simulink model "Modell_PADDELEC_RB_V4"  (R2020a)
settings: Solver=VariableStepAuto  StartTime=0.0  StopTime=250  RelTol=1e-3
values from neighbouring files (symbols this model uses):
  A_s = 3.5    [start.m]
  BAT = clsBattery    [start.m]
  BLDC = clsBLDC    [start.m]
  BoatHull = clsBoatHull    [start.m]
  c_r = 0.003    [start.m]
  MotorECU = clsMotorECU    [start.m]
libraries: fl_lib x54, nesl_utility x28, ee_lib x4, simulink x2, eeGeneralControl x1
settings Model: Creator=Rene Budich  LastModifiedBy=Rene Budich

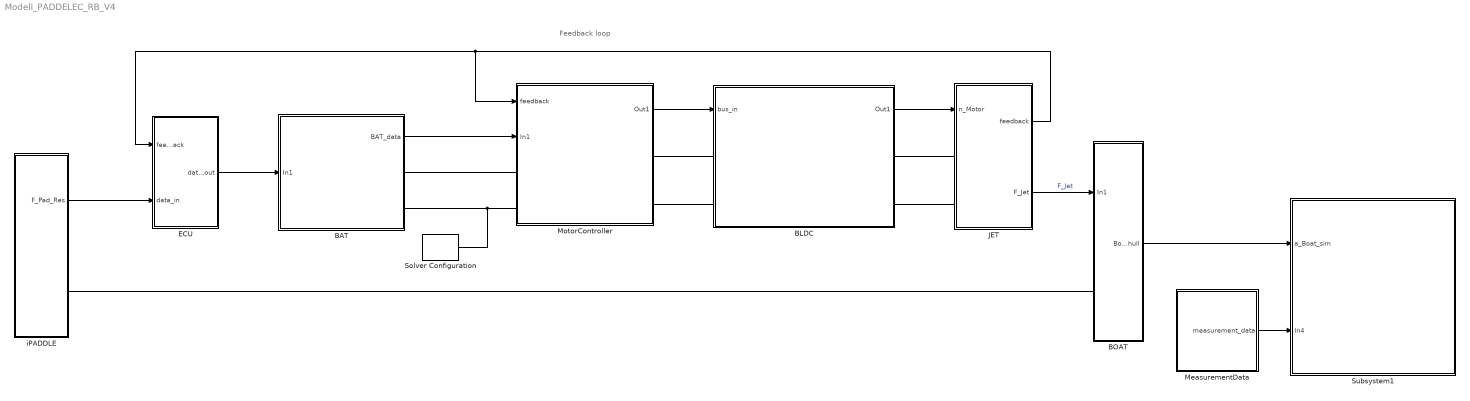
== system Modell_PADDELEC_RB_V4 ==
  note: Feedback loop
  BAT : Subsystem
      mask Display: image('Battery.jpg'); % Use "Edit Image" on toolstrip to change.
  BLDC : Subsystem
      mask Display: image('Motor.png'); % Use "Edit Image" on toolstrip to change.
  BOAT : Subsystem
  ECU : Subsystem
  "JET " : Subsystem
  MeasurementData : Subsystem
  MotorController : Subsystem
      mask Display: image('MotorECU.jpg'); % Use "Edit Image" on toolstrip to change.
  Solver Configuration : nesl_utility/Solver Configuration  PhysicalDomain=network_engine_domain  SubClassName=solver  LeftPortType=input  RightPortType=generic  Tones=[]  Harmonics=[]  SimulateNoise=off  Profile=off  UseLocalSampling=off  EnableSwitchedLinearOptims=on  FrequencyDomain=off  UseCCode=off  RelTol=0.001  AbsTol=1e-06  MinStep=1e-09  ToWorkspace=off  RevertToSquareIcSolve=off  NumHomotopyIterations=100  PhasorMode=off  PhasorModeNumHarmonics=1  DoDC=off  ResidualTolerance=1e-09  UseLocalSolver=off  LocalSolverChoice=NE_BACKWARD_EULER_ADVANCER  LocalSolverSampleTime=0.001  DoFixedCost=off  MaxNonlinIter=3  MaxModeIter=2  LinearAlgebra=Sparse  EquationFormulation=NE_TIME_EF  DelaysMemoryBudget=1024  AutomaticFiltering=on  FilteringTimeConstant=0.001  PartitionStorageMethod=AS_NEEDED  PartitionMemoryBudget=1024  PartitionMethod=FAST
  Subsystem1 : Subsystem
  iPADDLE : Subsystem
  wires:
  MotorController/1(Out1) -> BLDC/1(bus_in)
  "JET "/2(F_Jet) -> BOAT/1(In1)  "F_Jet"
  iPADDLE/1(F_Pad_Res) -> ECU/2(data_in)
  ECU/1(data_out) -> BAT/1(In1)
  BOAT/1(Boat_hull) -> Subsystem1/1(a_Boat_sim)
  BAT/1(BAT_data) -> MotorController/2(In1)
  MeasurementData/1(measurement_data) -> Subsystem1/2(In4)
  BLDC/1(Out1) -> "JET "/1(n_Motor)
  "JET "/1(feedback) -> MotorController/1(feedback), ECU/1(feedback)
  connections:
  MotorController/LConn2 -- Solver Configuration/RConn1 -- BAT/RConn2
  MotorController/LConn1 -- BAT/RConn1
  BLDC/LConn2 -- MotorController/RConn2
  BLDC/LConn1 -- MotorController/RConn1
  iPADDLE/RConn1 -- BOAT/LConn1
  BLDC/RConn1 -- "JET "/LConn1
  BLDC/RConn2 -- "JET "/LConn2

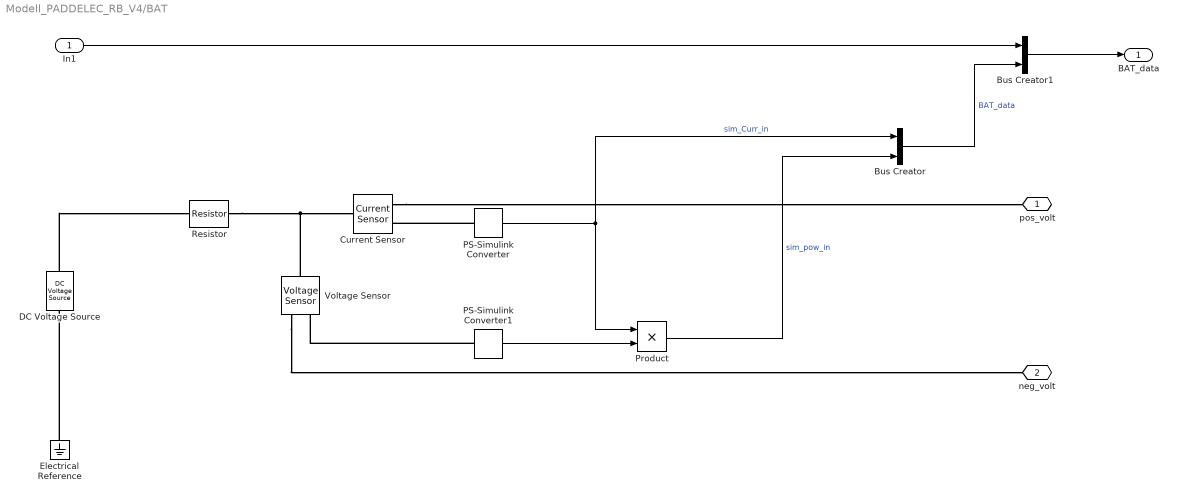
== system Modell_PADDELEC_RB_V4/BAT ==
  In1 : Inport
  Bus Creator : BusCreator  Inputs=2
  Bus Creator1 : BusCreator  Inputs=2
  Current Sensor : fl_lib/Electrical/Electrical Sensors/Current Sensor
  DC Voltage Source : fl_lib/Electrical/Electrical Sources/DC Voltage Source  v0=BAT.Voltage V
  Electrical Reference : fl_lib/Electrical/Electrical Elements/Electrical Reference
  PS-Simulink Converter : nesl_utility/PS-Simulink Converter  PhysicalDomain=network_engine_domain  SubClassName=ps_output  LeftPortType=input  RightPortType=output  PseudoPeriodic=off  Frequencies=[]  Unit=1  AffineConversion=off
  PS-Simulink Converter1 : nesl_utility/PS-Simulink Converter  PhysicalDomain=network_engine_domain  SubClassName=ps_output  LeftPortType=input  RightPortType=output  PseudoPeriodic=off  Frequencies=[]  Unit=1  AffineConversion=off
  Product : Product
  Resistor : fl_lib/Electrical/Electrical Elements/Resistor  R=BAT.InternalResistance Ohm  i_specify=off  i_priority=High  i=0 A  i_nominal_specify=off  i_nominal_unit=A  i_nominal_value=1  v_specify=off  v_priority=High  v=0 V  v_nominal_specify=off  v_nominal_unit=V  v_nominal_value=1
  Voltage Sensor : fl_lib/Electrical/Electrical Sensors/Voltage Sensor
  pos_volt : PMIOPort  Side=Right
  neg_volt : PMIOPort  Port=2  Side=Right
  BAT_data : Outport
  wires:
  PS-Simulink Converter/1 -> Product/1, Bus Creator/1  "sim_Curr_in"
  Product/1 -> Bus Creator/2  "sim_pow_in"
  PS-Simulink Converter1/1 -> Product/2
  Bus Creator1/1 -> BAT_data/1
  Bus Creator/1 -> Bus Creator1/2  "BAT_data"
  In1/1 -> Bus Creator1/1
  connections:
  Electrical Reference/LConn1 -- DC Voltage Source/RConn1
  Voltage Sensor/LConn1 -- Current Sensor/LConn1 -- Resistor/RConn1
  PS-Simulink Converter1/LConn1 -- Voltage Sensor/RConn1
  PS-Simulink Converter/LConn1 -- Current Sensor/RConn1
  DC Voltage Source/LConn1 -- Resistor/LConn1
  Voltage Sensor/RConn2 -- neg_volt/RConn1
  Current Sensor/RConn2 -- pos_volt/RConn1

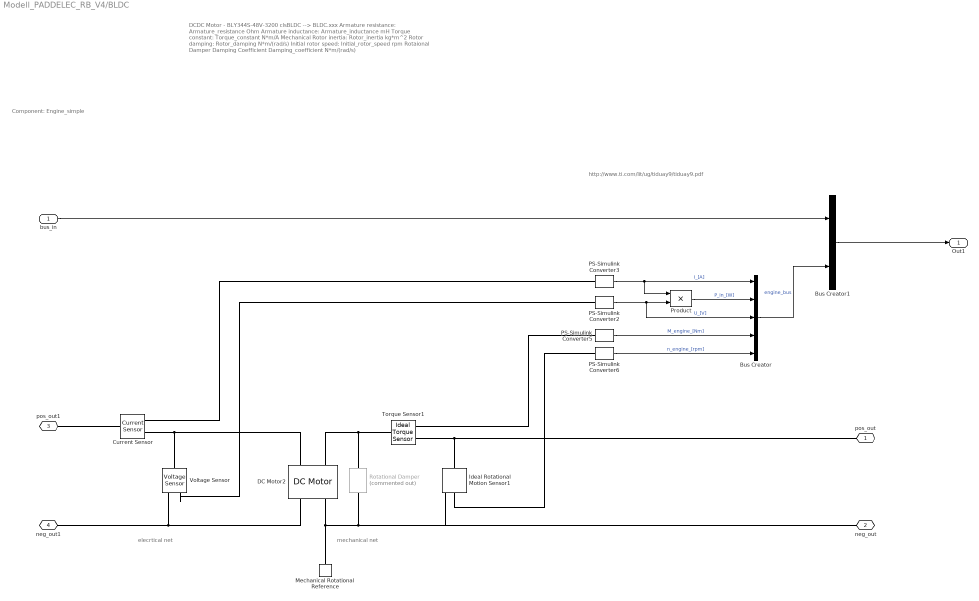
== system Modell_PADDELEC_RB_V4/BLDC ==
  note: http://www.ti.com/lit/ug/tiduay9/tiduay9.pdf
  note: mechanical net
  note: DCDC Motor - BLY344S-48V-3200
      |
      | clsBLDC --> BLDC.xxx
      |
      | Armature resistance:
      | Armature_resistance
      | Ohm
      |
      | Armature inductance:
      | Armature_inductance
      | mH
      |
      | Torque constant:
      | Torque_constant
      | N*m/A
      |
      | Mechanical
      |
      | Rotor inertia:
      | Rotor_inertia
      | kg*m^2
      |
      | Rotor damping:
      | Rotor_damping
      | N*m/(rad/s)
      |
      | Initial rotor speed:
      | Initial_rotor_speed
      | rpm
      |
      | Rotaional Damper
      |
      | Damping Coefficient
      | Damping_coefficient
      | N*m/(rad/s)
  note: elecrtical net
  note: Component:
      | Engine_simple
  bus_in : Inport
  Bus Creator : BusCreator  Inputs=5
  Bus Creator1 : BusCreator  Inputs=2
  Current Sensor : fl_lib/Electrical/Electrical Sensors/Current Sensor
  DC Motor2 : ee_lib/Electromechanical/Brushed Motors/DC Motor  field_option=ee.enum.field_option.pm  Rf=100 Ohm  Lf=1 H  Laf=0.15 H  If0=0 A  parameterization=1  Ra=BLDC.Armature_resistance Ohm  La=BLDC.Armature_inductance mH  emf_or_torque=2  Kv=0.00907 V/rpm  Ki=BLDC.Torque_constant N*m/A  T_stall=3e-3*4000/(2*pi*6.25) N*m  w_max=3200 rpm  w_rated=3200 rpm  P_rated=660 W  V_rated=48 V  J="BLDC.Rotor_inertia  kg*m^2"  lam_param=1  lam=BLDC.Rotor_damping N*m/(rad/s)  i_noload=0 A  V_i_noload=1.5 V  speed0=BLDC.Initial_rotor_speed rpm  alpha=3.93e-3 1/K  Tmeas=25 degC  thermal_mass=100 J/K  initial_temperature=25 degC
  Ideal Rotational Motion Sensor1 : fl_lib/Mechanical/Mechanical Sensors/Ideal Rotational Motion Sensor  wrap_angle=simscape.enum.onoff.off  offset=0 rad
  Mechanical Rotational Reference : fl_lib/Mechanical/Rotational Elements/Mechanical Rotational Reference
  PS-Simulink Converter2 : nesl_utility/PS-Simulink Converter  PhysicalDomain=network_engine_domain  SubClassName=ps_output  LeftPortType=input  RightPortType=output  PseudoPeriodic=off  Frequencies=[]  Unit=V  AffineConversion=off
  PS-Simulink Converter3 : nesl_utility/PS-Simulink Converter  PhysicalDomain=network_engine_domain  SubClassName=ps_output  LeftPortType=input  RightPortType=output  PseudoPeriodic=off  Frequencies=[]  Unit=A  AffineConversion=off
  PS-Simulink Converter5 : nesl_utility/PS-Simulink Converter  PhysicalDomain=network_engine_domain  SubClassName=ps_output  LeftPortType=input  RightPortType=output  PseudoPeriodic=off  Frequencies=[]  Unit=N*m  AffineConversion=on
  PS-Simulink Converter6 : nesl_utility/PS-Simulink Converter  PhysicalDomain=network_engine_domain  SubClassName=ps_output  LeftPortType=input  RightPortType=output  PseudoPeriodic=off  Frequencies=[]  Unit=rpm  AffineConversion=on
  Product : Product
  Rotational Damper : fl_lib/Mechanical/Rotational Elements/Rotational Damper  Commented=on  D=2.5000e-04 N*m/(rad/s)  w_specify=off  w_priority=High  w=0 rad/s  w_nominal_specify=off  w_nominal_unit=rad/s  w_nominal_value=1  t_specify=off  t_priority=High  t=0 N*m  t_nominal_specify=off  t_nominal_unit=N*m  t_nominal_value=1
  Torque Sensor1 : fl_lib/Mechanical/Mechanical Sensors/Ideal Torque Sensor
  Voltage Sensor : fl_lib/Electrical/Electrical Sensors/Voltage Sensor
  pos_out : PMIOPort  Side=Right
  neg_out : PMIOPort  Port=2  Side=Right
  pos_out1 : PMIOPort  Port=3  Side=Left
  neg_out1 : PMIOPort  Port=4  Side=Left
  Out1 : Outport
  wires:
  Bus Creator1/1 -> Out1/1
  bus_in/1 -> Bus Creator1/1
  Product/1 -> Bus Creator/2  "P_in_[W]"
  PS-Simulink Converter3/1 -> Bus Creator/1, Product/1  "I_[A]"
  PS-Simulink Converter2/1 -> Bus Creator/3, Product/2  "U_[V]"
  Bus Creator/1 -> Bus Creator1/2  "engine_bus"
  PS-Simulink Converter5/1 -> Bus Creator/4  "M_engine_[Nm]"
  PS-Simulink Converter6/1 -> Bus Creator/5  "n_engine_[rpm]"
  connections:
  DC Motor2/RConn1 -- Voltage Sensor/RConn2 -- neg_out1/RConn1
  Torque Sensor1/RConn1 -- Ideal Rotational Motion Sensor1/LConn1 -- pos_out/RConn1
  DC Motor2/RConn2 -- Rotational Damper/RConn1 -- neg_out/RConn1 -- Ideal Rotational Motion Sensor1/RConn1 -- Mechanical Rotational Reference/LConn1
  DC Motor2/LConn2 -- Torque Sensor1/LConn1 -- Rotational Damper/LConn1
  DC Motor2/LConn1 -- Current Sensor/RConn2 -- Voltage Sensor/LConn1
  Ideal Rotational Motion Sensor1/RConn2 -- PS-Simulink Converter6/LConn1
  Torque Sensor1/RConn2 -- PS-Simulink Converter5/LConn1
  pos_out1/RConn1 -- Current Sensor/LConn1
  Voltage Sensor/RConn1 -- PS-Simulink Converter2/LConn1
  Current Sensor/RConn1 -- PS-Simulink Converter3/LConn1

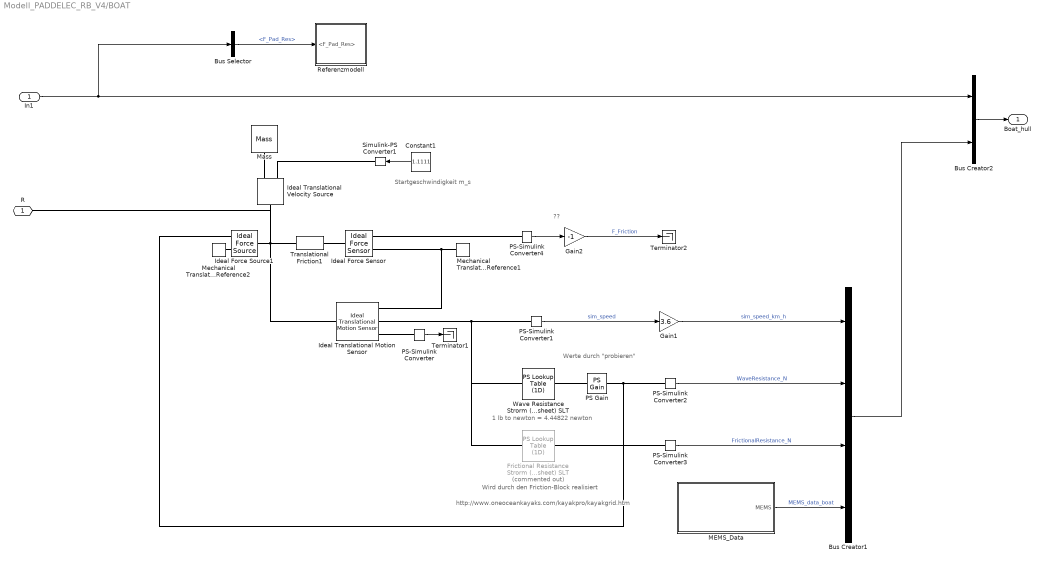
== system Modell_PADDELEC_RB_V4/BOAT ==
  note: ??
  note: Startgeschwindigkeit m_s
  note: Wird durch den Friction-Block realisiert
  note: 1 lb to newton = 4.44822 newton
  note: http://www.oneoceankayaks.com/kayakpro/kayakgrid.htm
  note: Werte durch "probieren"
  In1 : Inport
  Bus Creator1 : BusCreator  Inputs=4
  Bus Creator2 : BusCreator  Inputs=2
  Bus Selector : BusSelector  OutputSignals=signal1.controller.signal1.signal1.paddle.F_Pad_Res
  Constant1 : Constant  Value=1.1111
  Frictional Resistance Strorm (datasheet) SLT : fl_lib/Physical Signals/Lookup Tables/PS Lookup Table (1D)  Commented=on  x=SpeedVec_m_s m/s  f=FricResistance_N  interp_method=simscape.enum.interpolation.smooth  extrap_method=simscape.enum.extrapolation.linear
      settings: SourceProductBaseCode=SS
  Gain1 : Gain  Gain=3.6
  Gain2 : Gain  Gain=-1
  Ideal Force Sensor : fl_lib/Mechanical/Mechanical Sensors/Ideal Force Sensor
  Ideal Force Source1 : fl_lib/Mechanical/Mechanical Sources/Ideal Force Source
  Ideal Translational Motion Sensor : fl_lib/Mechanical/Mechanical Sensors/Ideal Translational Motion Sensor  offset=0 m
  Ideal Translational Velocity Source : fl_lib/Mechanical/Mechanical Sources/Ideal Translational Velocity Source
  MEMS_Data : Subsystem
      mask Display: image('D:\00_Sandbox\Matlab\Modell_20200324\03_symbols\Lagesensoren.png'); % Use "Edit Image" on toolstrip to change.
  Mass : fl_lib/Mechanical/Translational Elements/Mass  mass=BoatHull.Mass + 195.5 kg  v_specify=off  v_priority=High  v=0 m/s  v_nominal_specify=off  v_nominal_unit=m/s  v_nominal_value=1  f_specify=off  f_priority=None  f=0 N  f_nominal_specify=off  f_nominal_unit=N  f_nominal_value=1
  Mechanical Translational Reference1 : fl_lib/Mechanical/Translational Elements/Mechanical Translational Reference
  Mechanical Translational Reference2 : fl_lib/Mechanical/Translational Elements/Mechanical Translational Reference
  PS Gain : fl_lib/Physical Signals/Functions/PS Gain  gain=-32
  PS-Simulink Converter : nesl_utility/PS-Simulink Converter  PhysicalDomain=network_engine_domain  SubClassName=ps_output  LeftPortType=input  RightPortType=output  PseudoPeriodic=off  Frequencies=[]  Unit=inherit  AffineConversion=off
  PS-Simulink Converter1 : nesl_utility/PS-Simulink Converter  PhysicalDomain=network_engine_domain  SubClassName=ps_output  LeftPortType=input  RightPortType=output  PseudoPeriodic=off  Frequencies=[]  Unit=inherit  AffineConversion=off
  PS-Simulink Converter2 : nesl_utility/PS-Simulink Converter  PhysicalDomain=network_engine_domain  SubClassName=ps_output  LeftPortType=input  RightPortType=output  PseudoPeriodic=off  Frequencies=[]  Unit=inherit  AffineConversion=on
  PS-Simulink Converter3 : nesl_utility/PS-Simulink Converter  PhysicalDomain=network_engine_domain  SubClassName=ps_output  LeftPortType=input  RightPortType=output  PseudoPeriodic=off  Frequencies=[]  Unit=inherit  AffineConversion=on
  PS-Simulink Converter4 : nesl_utility/PS-Simulink Converter  PhysicalDomain=network_engine_domain  SubClassName=ps_output  LeftPortType=input  RightPortType=output  PseudoPeriodic=off  Frequencies=[]  Unit=inherit  AffineConversion=off
  Referenzmodell : Subsystem
  Simulink-PS Converter1 : nesl_utility/Simulink-PS Converter  PhysicalDomain=network_engine_domain  SubClassName=ps_input  LeftPortType=input  RightPortType=output  PseudoPeriodic=off  Frequencies=[]  NoiseDistribution=none  NoiseParameters=[]  Unit=1  AffineConversion=off  FilteringAndDerivatives=provide  SimscapeFilterOrder=1  InputFilterTimeConstant=0.001  UdotUserProvided=0
  Terminator1 : Terminator
  Terminator2 : Terminator
  Translational Friction1 : fl_lib/Mechanical/Translational Elements/Translational Friction  brkwy_frc=BoatHull.BreakawayFrictionForce N  brkwy_vel=BoatHull.BreakawayFrictionVelocity m/s  Col_frc=BoatHull.ColumbFrictionForce N  visc_coef=BoatHull.ViscousFriction N/(m/s)  v_specify=off  v_priority=None  v=0 m/s  v_nominal_specify=off  v_nominal_unit=m/s  v_nominal_value=1  f_specify=off  f_priority=None  f=0 N  f_nominal_specify=off  f_nominal_unit=N  f_nominal_value=1
      settings: SourceProductBaseCode=SS  InternalSimscapePortConfiguration="{\"Bottom\":[],\"Left\":[{\"id\":\"R\",\"label\":\"R\",\"type\":\"foundation.mechanical.translational.translational\"}],\"Right\":[{\"id\":\"C\",\"label\":\"C\",\"type\":\"foundation.mechanical.translational.translational\"}],\"Top\":[]}"
  Wave Resistance Strorm (datasheet) SLT : fl_lib/Physical Signals/Lookup Tables/PS Lookup Table (1D)  x=BoatHull.SpeedVec_m_s m/s  f=BoatHull.WaveResistance_N  interp_method=simscape.enum.interpolation.smooth  extrap_method=simscape.enum.extrapolation.linear
      settings: SourceProductBaseCode=SS
  R : PMIOPort  Side=Left
  Boat_hull : Outport  VectorParamsAs1DForOutWhenUnconnected=off
  wires:
  PS-Simulink Converter/1 -> Terminator1/1
  PS-Simulink Converter2/1 -> Bus Creator1/2  "WaveResistance_N"
  Gain1/1 -> Bus Creator1/1  "sim_speed_km_h"
  PS-Simulink Converter1/1 -> Gain1/1  "sim_speed"
  PS-Simulink Converter3/1 -> Bus Creator1/3  "FrictionalResistance_N"
  PS-Simulink Converter4/1 -> Gain2/1
  Constant1/1 -> Simulink-PS Converter1/1
  MEMS_Data/1(MEMS) -> Bus Creator1/4  "MEMS_data_boat"
  In1/1 -> Bus Selector/1, Bus Creator2/1
  Bus Creator1/1 -> Bus Creator2/2
  Bus Creator2/1 -> Boat_hull/1
  Gain2/1 -> Terminator2/1  "F_Friction"
  Bus Selector/1 -> Referenzmodell/1(<F_Pad_Res>)  "<F_Pad_Res>"
  connections:
  Ideal Translational Motion Sensor/LConn1 -- R/RConn1 -- Ideal Translational Velocity Source/LConn1 -- Ideal Force Source1/LConn1 -- Translational Friction1/LConn1
  Ideal Translational Motion Sensor/RConn1 -- Mechanical Translational Reference1/LConn1 -- Ideal Force Sensor/RConn1
  PS-Simulink Converter/LConn1 -- Ideal Translational Motion Sensor/RConn3
  Ideal Translational Motion Sensor/RConn2 -- Frictional Resistance Strorm (datasheet) SLT/LConn1 -- Wave Resistance Strorm (datasheet) SLT/LConn1 -- PS-Simulink Converter1/LConn1
  PS-Simulink Converter3/LConn1 -- Frictional Resistance Strorm (datasheet) SLT/RConn1
  PS-Simulink Converter2/LConn1 -- Ideal Force Source1/RConn1 -- PS Gain/RConn1
  PS Gain/LConn1 -- Wave Resistance Strorm (datasheet) SLT/RConn1
  PS-Simulink Converter4/LConn1 -- Ideal Force Sensor/RConn2
  Ideal Force Sensor/LConn1 -- Translational Friction1/RConn1
  Simulink-PS Converter1/RConn1 -- Ideal Translational Velocity Source/RConn1
  Ideal Translational Velocity Source/RConn2 -- Mass/LConn1
  Mechanical Translational Reference2/LConn1 -- Ideal Force Source1/RConn2

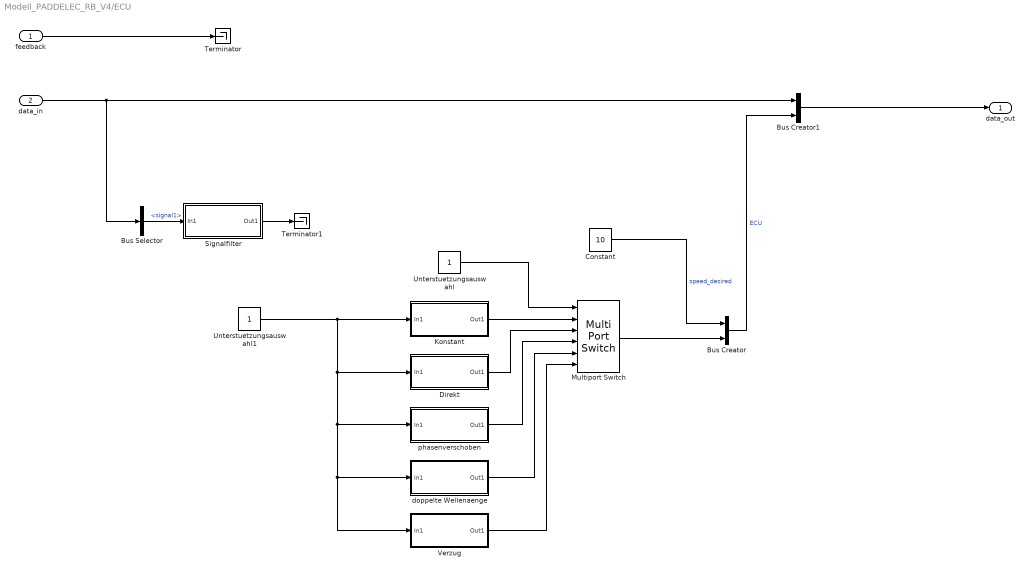
== system Modell_PADDELEC_RB_V4/ECU ==
  feedback : Inport
  data_in : Inport  Port=2
  Bus Creator : BusCreator  Inputs=2
  Bus Creator1 : BusCreator  Inputs=2
  Bus Selector : BusSelector  OutputSignals=MEMS_data_paddel.signal1
  Constant : Constant  Value=10
  Direkt : Subsystem
  Konstant : Subsystem
  Multiport Switch : MultiPortSwitch  Inputs=5
  Signalfilter : Subsystem
  Terminator : Terminator
  Terminator1 : Terminator
  Unterstuetzungsauswahl : Constant
  Unterstuetzungsauswahl1 : Constant
  Verzug : Subsystem
  doppelte Wellenaenge : Subsystem
  phasenverschoben : Subsystem
  data_out : Outport  VectorParamsAs1DForOutWhenUnconnected=off
  wires:
  Konstant/1(Out1) -> Multiport Switch/2
  Unterstuetzungsauswahl1/1 -> Verzug/1(In1), doppelte Wellenaenge/1(In1), phasenverschoben/1(In1), Direkt/1(In1), Konstant/1(In1)
  Direkt/1(Out1) -> Multiport Switch/3
  Unterstuetzungsauswahl/1 -> Multiport Switch/1
  phasenverschoben/1(Out1) -> Multiport Switch/4
  doppelte Wellenaenge/1(Out1) -> Multiport Switch/5
  Verzug/1(Out1) -> Multiport Switch/6
  Constant/1 -> Bus Creator/1  "speed_desired"
  Multiport Switch/1 -> Bus Creator/2
  data_in/1 -> Bus Creator1/1, Bus Selector/1
  Bus Selector/1 -> Signalfilter/1(In1)  "<signal1>"
  feedback/1 -> Terminator/1
  Bus Creator/1 -> Bus Creator1/2  "ECU"
  Bus Creator1/1 -> data_out/1
  Signalfilter/1(Out1) -> Terminator1/1

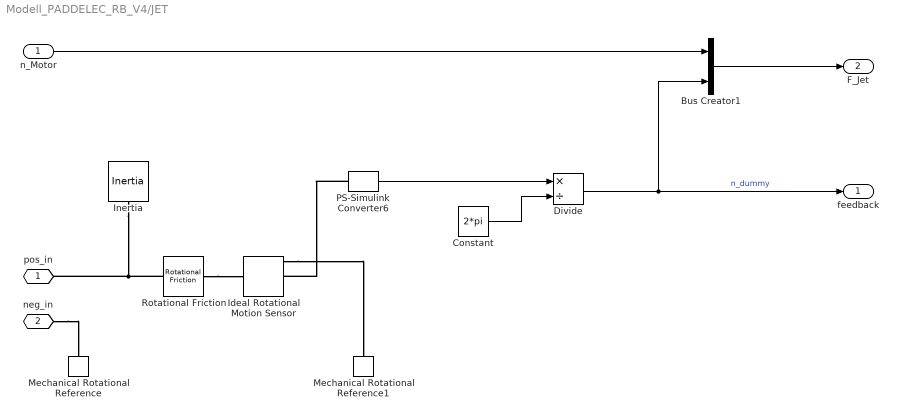
== system Modell_PADDELEC_RB_V4/JET  ==
  n_Motor : Inport
  Bus Creator1 : BusCreator  Inputs=2
  Constant : Constant  Value=2*pi
  Divide : Product  Inputs=*/
  Ideal Rotational Motion Sensor : fl_lib/Mechanical/Mechanical Sensors/Ideal Rotational Motion Sensor  wrap_angle=simscape.enum.onoff.off  offset=0 rad
  Inertia : fl_lib/Mechanical/Rotational Elements/Inertia  inertia=0.01 kg*m^2  w_specify=off  w_priority=High  w=0 rad/s  w_nominal_specify=off  w_nominal_unit=rad/s  w_nominal_value=1  t_specify=off  t_priority=None  t=0 N*m  t_nominal_specify=off  t_nominal_unit=N*m  t_nominal_value=1
  Mechanical Rotational Reference : fl_lib/Mechanical/Rotational Elements/Mechanical Rotational Reference
  Mechanical Rotational Reference1 : fl_lib/Mechanical/Rotational Elements/Mechanical Rotational Reference
  PS-Simulink Converter6 : nesl_utility/PS-Simulink Converter  PhysicalDomain=network_engine_domain  SubClassName=ps_output  LeftPortType=input  RightPortType=output  PseudoPeriodic=off  Frequencies=[]  Unit=rpm  AffineConversion=on
  Rotational Friction : fl_lib/Mechanical/Rotational Elements/Rotational Friction  brkwy_trq=10 N*m  brkwy_vel=0.1 rad/s  Col_trq=5 N*m  visc_coef=0.001 N*m/(rad/s)  w_specify=off  w_priority=None  w=0 rad/s  w_nominal_specify=off  w_nominal_unit=rad/s  w_nominal_value=1  t_specify=off  t_priority=None  t=0 N*m  t_nominal_specify=off  t_nominal_unit=N*m  t_nominal_value=1
  pos_in : PMIOPort  Side=Left
  neg_in : PMIOPort  Port=2  Side=Left
  feedback : Outport
  F_Jet : Outport  Port=2
  wires:
  Bus Creator1/1 -> F_Jet/1
  n_Motor/1 -> Bus Creator1/1
  PS-Simulink Converter6/1 -> Divide/1
  Constant/1 -> Divide/2
  Divide/1 -> feedback/1, Bus Creator1/2  "n_dummy"
  connections:
  Rotational Friction/LConn1 -- Inertia/LConn1 -- pos_in/RConn1
  neg_in/RConn1 -- Mechanical Rotational Reference/LConn1
  Ideal Rotational Motion Sensor/RConn1 -- Mechanical Rotational Reference1/LConn1
  Rotational Friction/RConn1 -- Ideal Rotational Motion Sensor/LConn1
  PS-Simulink Converter6/LConn1 -- Ideal Rotational Motion Sensor/RConn2

== system Modell_PADDELEC_RB_V4/MeasurementData ==
  Bus Creator : BusCreator  Inputs=2
  From Workspace1 : FromWorkspace  VariableName=tsc_paddel4.scaledAccelX
  From Workspace2 : FromWorkspace  VariableName=tsc_paddel4.speed
  Gain : Gain  Gain=-1
  Gain1 : Gain  Gain=3.6
  measurement_data : Outport
  wires:
  From Workspace1/1 -> Gain/1  "a_Boat"
  Gain/1 -> Bus Creator/1  "a_Boat"
  From Workspace2/1 -> Gain1/1  "v_Boat"
  Bus Creator/1 -> measurement_data/1
  Gain1/1 -> Bus Creator/2  "MEAS_v_Boat_km_h"

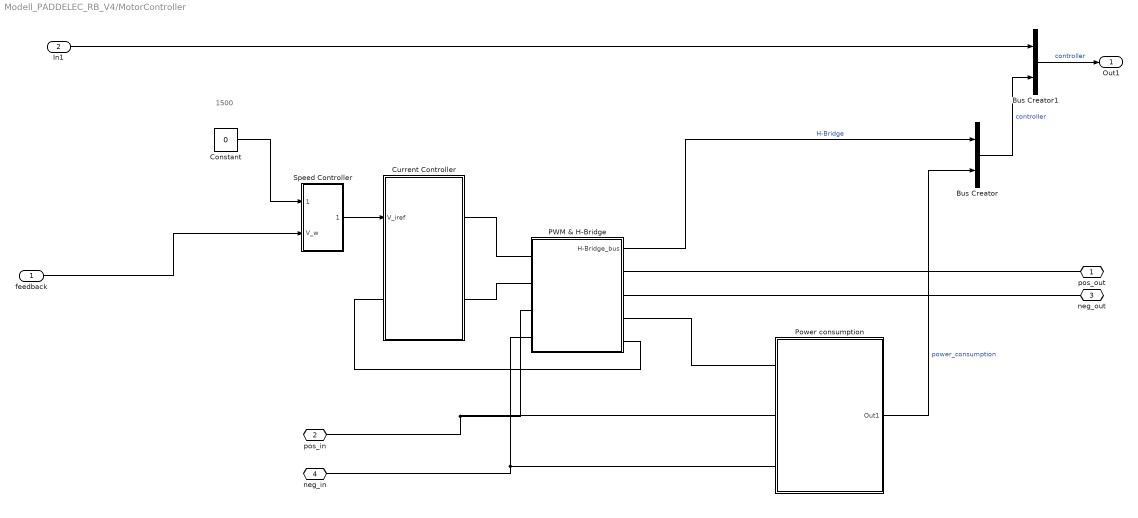
== system Modell_PADDELEC_RB_V4/MotorController ==
  note: 1500
  feedback : Inport
  In1 : Inport  Port=2
  Bus Creator : BusCreator  Inputs=2
  Bus Creator1 : BusCreator  Inputs=2
  Constant : Constant  Value=0
  Current Controller : Subsystem
  PWM & H-Bridge : Subsystem
  Power consumption : Subsystem
  Speed Controller : Subsystem  VariantControl=VSS_SpeedController_simple
  pos_out : PMIOPort  Side=Right
  pos_in : PMIOPort  Port=2  Side=Left
  neg_out : PMIOPort  Port=3  Side=Right
  neg_in : PMIOPort  Port=4  Side=Left
  Out1 : Outport
  wires:
  In1/1 -> Bus Creator1/1
  Power consumption/1(Out1) -> Bus Creator/2  "power_consumption"
  feedback/1 -> Speed Controller/2(V_w)
  Speed Controller/1(V_iref) -> Current Controller/1(V_iref)
  PWM & H-Bridge/1(H-Bridge_bus) -> Bus Creator/1  "H-Bridge"
  Bus Creator/1 -> Bus Creator1/2  "controller"
  Constant/1 -> Speed Controller/1(V_wref)
  Bus Creator1/1 -> Out1/1  "controller"
  connections:
  neg_out/RConn1 -- PWM & H-Bridge/RConn2
  PWM & H-Bridge/LConn1 -- Current Controller/RConn1
  Current Controller/RConn2 -- PWM & H-Bridge/LConn2
  pos_out/RConn1 -- PWM & H-Bridge/RConn1
  Power consumption/LConn1 -- PWM & H-Bridge/RConn3
  Current Controller/LConn1 -- PWM & H-Bridge/RConn4
  pos_in/RConn1 -- PWM & H-Bridge/LConn3 -- Power consumption/LConn2
  neg_in/RConn1 -- PWM & H-Bridge/LConn4 -- Power consumption/LConn3

== system Modell_PADDELEC_RB_V4/Subsystem1 ==
  a_Boat_sim : Inport
  In4 : Inport  Port=2
  Bus Selector : BusSelector  OutputSignals=signal2.sim_speed_km_h,signal2.WaveResistance_N
  Bus Selector1 : BusSelector  OutputSignals=a_Boat,MEAS_v_Boat_km_h
  v_Boat : Scope  NumInputPorts=2
  v_Boat1 : Scope  NumInputPorts=2
  wires:
  a_Boat_sim/1 -> Bus Selector/1
  In4/1 -> Bus Selector1/1
  Bus Selector/1 -> v_Boat/1  "<sim_speed_km_h>"
  Bus Selector/2 -> v_Boat/2  "<WaveResistance_N>"
  Bus Selector1/1 -> v_Boat1/1  "<a_Boat>"
  Bus Selector1/2 -> v_Boat1/2  "<MEAS_v_Boat_km_h>"

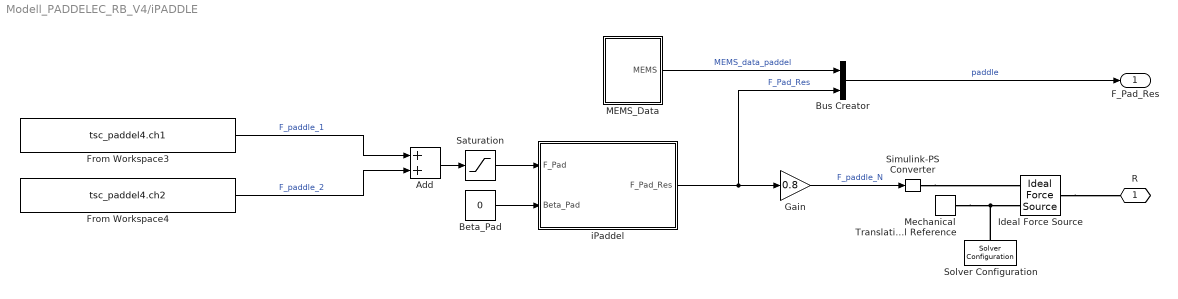
== system Modell_PADDELEC_RB_V4/iPADDLE ==
  Add : Sum
  Beta_Pad : Constant  Value=0
  Bus Creator : BusCreator  Inputs=2
  From Workspace3 : FromWorkspace  VariableName=tsc_paddel4.ch1
  From Workspace4 : FromWorkspace  VariableName=tsc_paddel4.ch2
  Gain : Gain  Gain=0.8
  Ideal Force Source : fl_lib/Mechanical/Mechanical Sources/Ideal Force Source
  MEMS_Data : Subsystem
  Mechanical Translational Reference : fl_lib/Mechanical/Translational Elements/Mechanical Translational Reference
  Saturation : Saturate  UpperLimit=inf  LowerLimit=0
  Simulink-PS Converter : nesl_utility/Simulink-PS Converter  PhysicalDomain=network_engine_domain  SubClassName=ps_input  LeftPortType=input  RightPortType=output  PseudoPeriodic=off  Frequencies=[]  NoiseDistribution=none  NoiseParameters=[]  Unit=1  AffineConversion=off  FilteringAndDerivatives=provide  SimscapeFilterOrder=1  InputFilterTimeConstant=0.001  UdotUserProvided=0
  Solver Configuration : nesl_utility/Solver Configuration  PhysicalDomain=network_engine_domain  SubClassName=solver  LeftPortType=input  RightPortType=generic  Tones=[]  Harmonics=[]  SimulateNoise=off  Profile=off  UseLocalSampling=off  EnableSwitchedLinearOptims=on  FrequencyDomain=off  UseCCode=off  RelTol=0.001  AbsTol=1e-06  MinStep=1e-09  ToWorkspace=off  RevertToSquareIcSolve=off  NumHomotopyIterations=100  PhasorMode=off  PhasorModeNumHarmonics=1  DoDC=off  ResidualTolerance=1e-09  UseLocalSolver=off  LocalSolverChoice=NE_BACKWARD_EULER_ADVANCER  LocalSolverSampleTime=0.001  DoFixedCost=off  MaxNonlinIter=3  MaxModeIter=2  LinearAlgebra=auto  EquationFormulation=NE_TIME_EF  DelaysMemoryBudget=1024  AutomaticFiltering=on  FilteringTimeConstant=0.001  PartitionStorageMethod=AS_NEEDED  PartitionMemoryBudget=1024  PartitionMethod=ROBUST
  iPaddel : Subsystem
  R : PMIOPort  Side=Right
  F_Pad_Res : Outport
  wires:
  Beta_Pad/1 -> iPaddel/2(Beta_Pad)
  Add/1 -> Saturation/1
  From Workspace3/1 -> Add/1  "F_paddle_1"
  From Workspace4/1 -> Add/2  "F_paddle_2"
  iPaddel/1(F_Pad_Res) -> Gain/1, Bus Creator/2  "F_Pad_Res"
  Saturation/1 -> iPaddel/1(F_Pad)
  Gain/1 -> Simulink-PS Converter/1  "F_paddle_N"
  MEMS_Data/1(MEMS) -> Bus Creator/1  "MEMS_data_paddel"
  Bus Creator/1 -> F_Pad_Res/1  "paddle"
  connections:
  Mechanical Translational Reference/LConn1 -- Solver Configuration/RConn1 -- Ideal Force Source/RConn2
  Simulink-PS Converter/RConn1 -- Ideal Force Source/RConn1
  Ideal Force Source/LConn1 -- R/RConn1

== system Modell_PADDELEC_RB_V4/BOAT/MEMS_Data ==
  Beta_Pad : Constant  Value=0
  Bus Creator : BusCreator  Inputs=1
  MEMS : Outport
  wires:
  Beta_Pad/1 -> Bus Creator/1
  Bus Creator/1 -> MEMS/1

== system Modell_PADDELEC_RB_V4/BOAT/Referenzmodell ==
  <F_Pad_Res> : Inport
  Delay : Delay
  Divide : Product  Inputs=*/
  Integrator : Integrator  InitialConditionSource=external
  Sum1 : Sum  Inputs=|+-
  Terminator3 : Terminator
  m_Boat : Constant  Value=BoatHull.Mass + 195.5
  resistances : Subsystem
  v_0 : Constant  SampleTime=-1
  wires:
  m_Boat/1 -> Divide/2
  Sum1/1 -> Divide/1
  Delay/1 -> resistances/1(v_Boat_In)
  Divide/1 -> Integrator/1
  Integrator/1 -> Terminator3/1, Delay/1  "v_Refernce_modell"
  v_0/1 -> Integrator/2
  resistances/1(F_Resis_Out) -> Sum1/2
  <F_Pad_Res>/1 -> Sum1/1

== system Modell_PADDELEC_RB_V4/ECU/Direkt ==
  In1 : Inport
  Out1 : Outport
  wires:
  In1/1 -> Out1/1

== system Modell_PADDELEC_RB_V4/ECU/Konstant ==
  In1 : Inport
  Moving Average : eeGeneralControl/Moving Average  VariantControl=Variant1  LabelModeActiveChoice=Continuous  f=0.08  x0=0  Ts=0
      settings: SourceProductBaseCode=PS
  Out1 : Outport
  wires:
  In1/1 -> Moving Average/1
  Moving Average/1 -> Out1/1

== system Modell_PADDELEC_RB_V4/ECU/Signalfilter ==
  In1 : Inport
  Out1 : Outport
  wires:
  In1/1 -> Out1/1

== system Modell_PADDELEC_RB_V4/ECU/Verzug ==
  In1 : Inport
  Out1 : Outport
  wires:
  In1/1 -> Out1/1

== system Modell_PADDELEC_RB_V4/ECU/doppelte Wellenaenge ==
  In1 : Inport
  Out1 : Outport
  wires:
  In1/1 -> Out1/1

== system Modell_PADDELEC_RB_V4/ECU/phasenverschoben ==
  In1 : Inport
  Out1 : Outport
  wires:
  In1/1 -> Out1/1

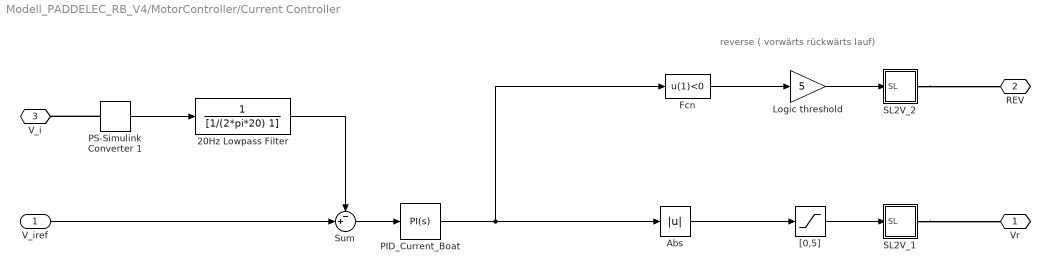
== system Modell_PADDELEC_RB_V4/MotorController/Current Controller ==
  note: reverse ( vorwärts rückwärts lauf)
  V_iref : Inport
  20Hz Lowpass Filter : TransferFcn  Denominator=[1/(2*pi*20) 1]
  Abs : Abs
  Fcn : Fcn  Expr=u(1)<0
  Logic threshold : Gain  Gain=5
  PID_Current_Boat : simulink/Continuous/PID Controller  Controller=PI  Form=Parallel  TimeDomain=Continuous-time  UseExternalTs=off  SampleTime=-1  IntegratorMethod=Forward Euler  FilterMethod=Forward Euler  ControllerParametersSource=internal  P=MotorECU.Current_Prop  I=MotorECU.Current_Int  D=0  UseFilter=on  N=100  TunerSelectOption=Transfer Function Based (PID Tuner App)  InitialConditionSource=internal  InitialConditionForIntegrator=0  InitialConditionForFilter=0  DifferentiatorICPrevScaledInput=0  ExternalReset=none  TrackingMode=off  Kt=1  LimitOutput=off  UpperSaturationLimit=1.71  LowerSaturationLimit=-5  LinearizeAsGain=on  AntiWindupMode=back-calculation  Kb=1  POutMin=[]  POutMax=[]  IOutMin=[]  IOutMax=[]  DOutMin=[]  DOutMax=[]  NOutMin=[]  NOutMax=[]  SumOutMin=[]  SumOutMax=[]  SaturationOutMin=[]  SaturationOutMax=[]  PParamMin=[]  PParamMax=[]  IParamMin=[]  IParamMax=[]  DParamMin=[]  DParamMax=[]  NParamMin=[]  NParamMax=[]  KbParamMin=[]  KbParamMax=[]  KtParamMin=[]  KtParamMax=[]  KbOutMin=[]  KbOutMax=[]  KtOutMin=[]  KtOutMax=[]  IntegratorOutMin=[]  IntegratorOutMax=[]  FilterOutMin=[]  FilterOutMax=[]  SumI1OutMin=[]  SumI1OutMax=[]  SumI2OutMin=[]  SumI2OutMax=[]  SumI3OutMin=[]  SumI3OutMax=[]  SumI4OutMin=[]  SumI4OutMax=[]  SumDOutMin=[]  SumDOutMax=[]  DifferentiatorOutMin=[]  DifferentiatorOutMax=[]  FilterDiffOutCoefMin=[]  FilterDiffOutCoefMax=[]  ReciprocalOutMin=[]  ReciprocalOutMax=[]  SumDenOutMin=[]  SumDenOutMax=[]  SumNumOutMin=[]  SumNumOutMax=[]  DivideOutMin=[]  DivideOutMax=[]  UdiffTsProdOutMin=[]  UdiffTsProdOutMax=[]  NTsProdOutMin=[]  NTsProdOutMax=[]  UintegralTsProdOutMin=[]  UintegralTsProdOutMax=[]  UngainTsProdOutMin=[]  UngainTsProdOutMax=[]  IntegratorContinuousStateAttributes=''  IntegratorStateMustResolveToSignalObject=off  IntegratorRTWStateStorageClass=Auto  FilterContinuousStateAttributes=''  FilterStateMustResolveToSignalObject=off  FilterRTWStateStorageClass=Auto  ParallelPVariant=InternalParameters  IdealPVariant=Disabled  IVariant=InternalParameters  DVariant=Disabled  IntegratorVariant=Continuous  SatVariant=Disabled  AWVariant=Passthrough  PCopyVariant=Disabled  TRVariant=Disabled  FdbkBlocksVariant=Forward  IdealPFdbkVariant=Disabled  SatFdbkVariant=Disabled  DerivativeFilterVariant=Disabled  NVariant=Disabled  NCopyVariant=Disabled_SignalSpec  FilterICVariant=Disabled  IntegratorICVariant=InternalICs  ExternalResetVariant=Disabled  TRSumVariant=Passthrough  SumFdbkVariant=Disabled  SumVariant=Sum_PI  TsampFilterVariant=InternalTs  TsampNgainVariant=Passthrough  TsampIntegralVariant=Passthrough
  PS-Simulink Converter 1 : nesl_utility/PS-Simulink Converter  PhysicalDomain=network_engine_domain  SubClassName=ps_output  LeftPortType=input  RightPortType=output  PseudoPeriodic=off  Frequencies=[]  Unit=A  AffineConversion=off
  SL2V_1 : Subsystem
  SL2V_2 : Subsystem
  Sum : Sum  Inputs=-+|
  "[0,5]" : Saturate  UpperLimit=5  LowerLimit=0
  Vr : PMIOPort  Side=Right
  REV : PMIOPort  Port=2  Side=Right
  V_i : PMIOPort  Port=3  Side=Left
  wires:
  "[0,5]"/1 -> SL2V_1/1(SL)
  Fcn/1 -> Logic threshold/1
  Abs/1 -> "[0,5]"/1
  20Hz Lowpass Filter/1 -> Sum/1
  V_iref/1 -> Sum/2
  Logic threshold/1 -> SL2V_2/1(SL)
  PID_Current_Boat/1 -> Fcn/1, Abs/1
  Sum/1 -> PID_Current_Boat/1
  PS-Simulink Converter 1/1 -> 20Hz Lowpass Filter/1
  connections:
  SL2V_2/RConn1 -- REV/RConn1
  SL2V_1/RConn1 -- Vr/RConn1
  PS-Simulink Converter 1/LConn1 -- V_i/RConn1

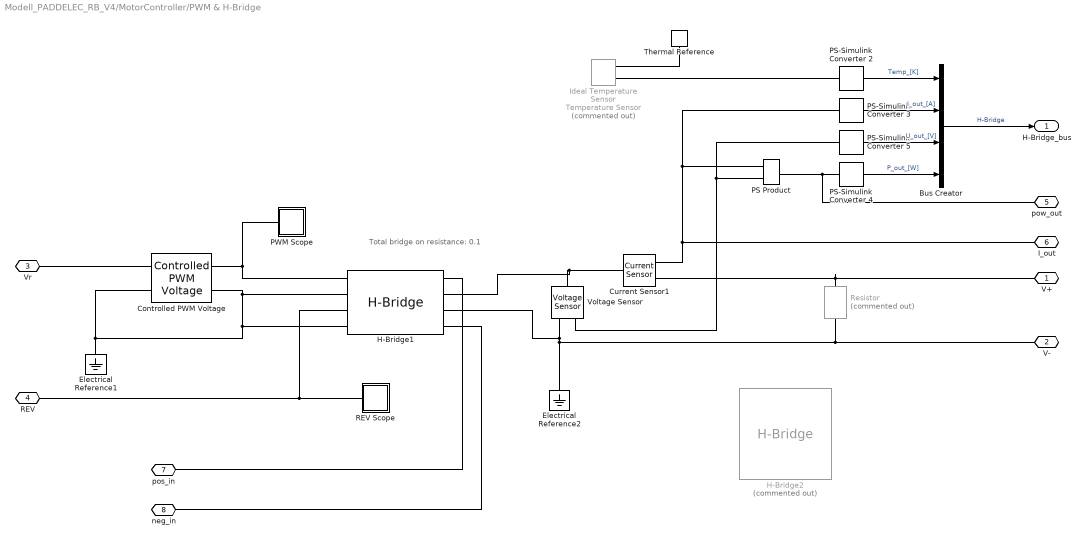
== system Modell_PADDELEC_RB_V4/MotorController/PWM & H-Bridge ==
  note: Total bridge on resistance: 0.1
  Bus Creator : BusCreator  Inputs=4
  Controlled PWM Voltage : ee_lib/Integrated Circuits/Controlled PWM Voltage  F=10000 Hz  TD=0 s  pulse_width_offset=0 s  pulse_min=0 s  Vmin=0 V  Vmax=5 V  Vm=5 V  pwm_or_av=2  event_type=1  sample_time=1e-6 s  u_min=0  u_max=1
  Current Sensor1 : fl_lib/Electrical/Electrical Sensors/Current Sensor
  Electrical Reference1 : fl_lib/Electrical/Electrical Elements/Electrical Reference
  Electrical Reference2 : fl_lib/Electrical/Electrical Elements/Electrical Reference
  H-Bridge1 : ee_lib/Semiconductors & Converters/Converters/H-Bridge  supply_ports=ee.enum.supply_ports.showsupply  Venable=2.5 V  Vmax=5.0 V  Vreverse=2.5 V  Vbrake=2.5 V  Vm=48 V  pwm_or_av=ee.enum.pwm_or_av.pwm  regenerative_braking_mode=ee.enum.converters.regenerative_braking_mode.depends_on_rev  discontinuous=ee.enum.current_profile.continuous  freewheeling_mode=ee.enum.converters.freewheeling_mode.one_switch_one_diode  Ron=0.1 Ohm  Don=0.05 Ohm  Goff=1e-6 S  Rload=10 Ohm  Lload=1e-5 H  F=10 kHz  thermal_mass=100 J/K  initial_temperature=298.15 K  Ron2=0.1 Ohm  Don2=0.05 Ohm  Tmeas=298.15 K  Tmeas2=398.15 K
      settings: InternalSimscapePortConfiguration="{\"Bottom\":[],\"Left\":[{\"id\":\"ENA\",\"label\":\"PWM\",\"type\":\"foundation.electrical.electrical\"},{\"id\":\"REF\",\"label\":\"REF\",\"type\":\"foundation.electrical.electrical\"},{\"id\":\"REV\",\"label\":\"REV\",\"type\":\"foundation.electrical.electrical\"},{\"id\":\"BRK\",\"label\":\"BRK\",\"type\":\"foundation.electrical.electrical\"}],\"Right\":[{\"id\":\"p1\",\"label\":\"V+\",\"type\":\"foundation.electrical.electrical\"},{\"id\":\"p2\",\"label\":\"+\",\"type\":\"foundation.electrical.electrical\"},{\"id\":\"n2\",\"label\":\"-\",\"type\":\"foundation.electrical.electrical\"},{\"id\":\"n1\",\"label\":\"V-\",\"type\":\"foundation.electrical.electrical\"}],\"Top\":[]}"
  H-Bridge2 : ee_lib/Semiconductors & Converters/Converters/H-Bridge  Commented=on  supply_ports=ee.enum.supply_ports.showsupply  Venable=2.5 V  Vmax=5 V  Vreverse=2.5 V  Vbrake=2.5 V  Vm=48 V  pwm_or_av=ee.enum.pwm_or_av.averaged  regenerative_braking_mode=ee.enum.converters.regenerative_braking_mode.always_enabled  discontinuous=ee.enum.current_profile.continuous  freewheeling_mode=ee.enum.converters.freewheeling_mode.one_switch_one_diode  Ron=0.1 Ohm  Don=0.1 Ohm  Goff=1e-6 S  Rload=10 Ohm  Lload=1e-5 H  F=10 kHz  thermal_mass=100 J/K  initial_temperature=298.15 K  Ron2=0.1 Ohm  Don2=0.05 Ohm  Tmeas=20 degC  Tmeas2=398.15 K
      settings: LogSimulationData=on  InternalSimscapePortConfiguration="{\"Bottom\":[],\"Left\":[{\"id\":\"ENA\",\"label\":\"PWM\",\"type\":\"foundation.electrical.electrical\"},{\"id\":\"REF\",\"label\":\"REF\",\"type\":\"foundation.electrical.electrical\"},{\"id\":\"REV\",\"label\":\"REV\",\"type\":\"foundation.electrical.electrical\"},{\"id\":\"BRK\",\"label\":\"BRK\",\"type\":\"foundation.electrical.electrical\"}],\"Right\":[{\"id\":\"p1\",\"label\":\"V+\",\"type\":\"foundation.electrical.electrical\"},{\"id\":\"p2\",\"label\":\"+\",\"type\":\"foundation.electrical.electrical\"},{\"id\":\"n2\",\"label\":\"-\",\"type\":\"foundation.electrical.electrical\"},{\"id\":\"n1\",\"label\":\"V-\",\"type\":\"foundation.electrical.electrical\"},{\"id\":\"H\",\"label\":\"H\",\"type\":\"foundation.thermal.thermal\"}],\"Top\":[]}"
  Ideal Temperature Sensor : fl_lib/Thermal/Thermal Sensors/Temperature Sensor  Commented=on
  PS Product : fl_lib/Physical Signals/Functions/PS Product
  PS-Simulink Converter 2 : nesl_utility/PS-Simulink Converter  PhysicalDomain=network_engine_domain  SubClassName=ps_output  LeftPortType=input  RightPortType=output  PseudoPeriodic=off  Frequencies=[]  Unit=K  AffineConversion=off
  PS-Simulink Converter 3 : nesl_utility/PS-Simulink Converter  PhysicalDomain=network_engine_domain  SubClassName=ps_output  LeftPortType=input  RightPortType=output  PseudoPeriodic=off  Frequencies=[]  Unit=A  AffineConversion=off
  PS-Simulink Converter 4 : nesl_utility/PS-Simulink Converter  PhysicalDomain=network_engine_domain  SubClassName=ps_output  LeftPortType=input  RightPortType=output  PseudoPeriodic=off  Frequencies=[]  Unit=W  AffineConversion=off
  PS-Simulink Converter 5 : nesl_utility/PS-Simulink Converter  PhysicalDomain=network_engine_domain  SubClassName=ps_output  LeftPortType=input  RightPortType=output  PseudoPeriodic=off  Frequencies=[]  Unit=V  AffineConversion=off
  PWM Scope : Subsystem
  REV Scope : Subsystem
  Resistor : fl_lib/Electrical/Electrical Elements/Resistor  Commented=on  R=10 kOhm  i_specify=off  i_priority=None  i=0 A  i_nominal_specify=off  i_nominal_unit=A  i_nominal_value=1  v_specify=off  v_priority=None  v=0 V  v_nominal_specify=off  v_nominal_unit=V  v_nominal_value=1
  Thermal Reference : fl_lib/Thermal/Thermal Elements/Thermal Reference
  Voltage Sensor : fl_lib/Electrical/Electrical Sensors/Voltage Sensor
  V+ : PMIOPort  Side=Right
  V- : PMIOPort  Port=2  Side=Right
  Vr : PMIOPort  Port=3  Side=Left
  REV : PMIOPort  Port=4  Side=Left
  pow_out : PMIOPort  Port=5  Side=Right
  I_out : PMIOPort  Port=6  Side=Right
  pos_in : PMIOPort  Port=7  Side=Left
  neg_in : PMIOPort  Port=8  Side=Left
  H-Bridge_bus : Outport
  wires:
  PS-Simulink Converter 2/1 -> Bus Creator/1  "Temp_[K]"
  Bus Creator/1 -> H-Bridge_bus/1  "H-Bridge"
  PS-Simulink Converter 3/1 -> Bus Creator/2  "I_out_[A]"
  PS-Simulink Converter 5/1 -> Bus Creator/3  "U_out_[V]"
  PS-Simulink Converter 4/1 -> Bus Creator/4  "P_out_[W]"
  connections:
  REV/RConn1 -- H-Bridge1/LConn3 -- REV Scope/LConn1
  Vr/RConn1 -- Controlled PWM Voltage/LConn1
  Electrical Reference1/LConn1 -- Controlled PWM Voltage/RConn2 -- H-Bridge1/LConn2 -- H-Bridge1/LConn4 -- Controlled PWM Voltage/LConn2
  PWM Scope/LConn1 -- H-Bridge1/LConn1 -- Controlled PWM Voltage/RConn1
  Voltage Sensor/RConn2 -- H-Bridge1/RConn3 -- Resistor/RConn1 -- V-/RConn1 -- Electrical Reference2/LConn1
  Voltage Sensor/LConn1 -- H-Bridge1/RConn2 -- Current Sensor1/LConn1
  PS-Simulink Converter 2/LConn1 -- Ideal Temperature Sensor/RConn2
  Thermal Reference/LConn1 -- Ideal Temperature Sensor/RConn1
  PS Product/LConn2 -- PS-Simulink Converter 5/LConn1 -- Voltage Sensor/RConn1
  Current Sensor1/RConn2 -- Resistor/LConn1 -- V+/RConn1
  Current Sensor1/RConn1 -- PS-Simulink Converter 3/LConn1 -- PS Product/LConn1 -- I_out/RConn1
  pow_out/RConn1 -- PS Product/RConn1 -- PS-Simulink Converter 4/LConn1
  pos_in/RConn1 -- H-Bridge1/RConn1
  neg_in/RConn1 -- H-Bridge1/RConn4

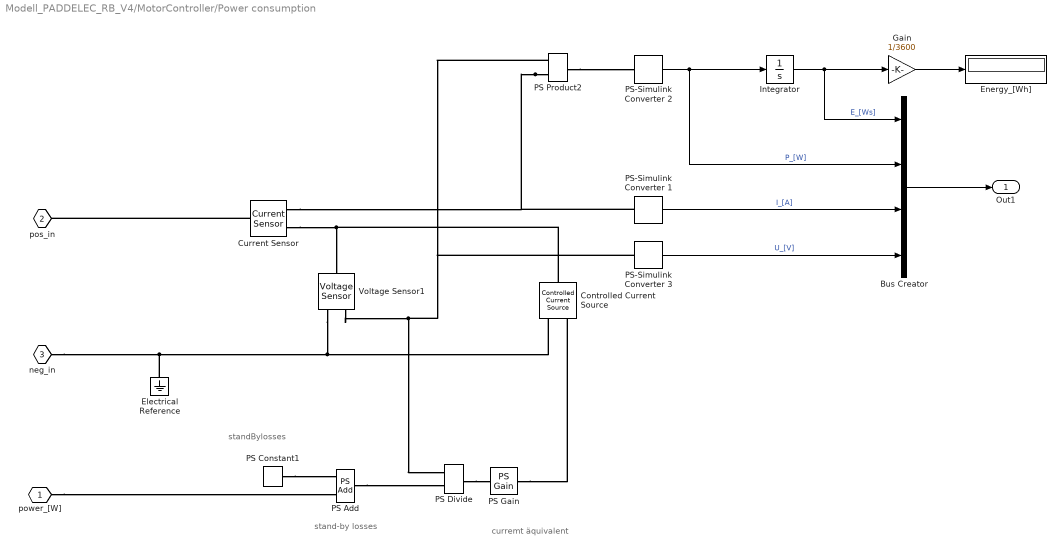
== system Modell_PADDELEC_RB_V4/MotorController/Power consumption ==
  note: standBylosses
  note: curremt äquivalent
  note: stand-by losses
  Bus Creator : BusCreator  Inputs=4
  Controlled Current Source : fl_lib/Electrical/Electrical Sources/Controlled Current Source
      settings: LogSimulationData=on
  Current Sensor : fl_lib/Electrical/Electrical Sensors/Current Sensor
  Electrical Reference : fl_lib/Electrical/Electrical Elements/Electrical Reference
  Energy_[Wh] : Display
  Gain : Gain  Gain=1/3600
  Integrator : Integrator
  PS Add : fl_lib/Physical Signals/Functions/PS Add
  PS Constant1 : fl_lib/Physical Signals/Sources/PS Constant  constant=MotorECU.stand_by_losses W
  PS Divide : fl_lib/Physical Signals/Functions/PS Divide
      settings: SourceProductBaseCode=SS
  PS Gain : fl_lib/Physical Signals/Functions/PS Gain  gain=-1
  PS Product2 : fl_lib/Physical Signals/Functions/PS Product
  PS-Simulink Converter 1 : nesl_utility/PS-Simulink Converter  PhysicalDomain=network_engine_domain  SubClassName=ps_output  LeftPortType=input  RightPortType=output  PseudoPeriodic=off  Frequencies=[]  Unit=A  AffineConversion=off
  PS-Simulink Converter 2 : nesl_utility/PS-Simulink Converter  PhysicalDomain=network_engine_domain  SubClassName=ps_output  LeftPortType=input  RightPortType=output  PseudoPeriodic=off  Frequencies=[]  Unit=W  AffineConversion=off
  PS-Simulink Converter 3 : nesl_utility/PS-Simulink Converter  PhysicalDomain=network_engine_domain  SubClassName=ps_output  LeftPortType=input  RightPortType=output  PseudoPeriodic=off  Frequencies=[]  Unit=V  AffineConversion=off
  Voltage Sensor1 : fl_lib/Electrical/Electrical Sensors/Voltage Sensor
  power_[W] : PMIOPort  Side=Left
  pos_in : PMIOPort  Port=2  Side=Left
  neg_in : PMIOPort  Port=3  Side=Left
  Out1 : Outport
  wires:
  PS-Simulink Converter 2/1 -> Integrator/1, Bus Creator/2  "P_[W]"
  Integrator/1 -> Gain/1, Bus Creator/1  "E_[Ws]"
  Bus Creator/1 -> Out1/1
  PS-Simulink Converter 3/1 -> Bus Creator/4  "U_[V]"
  PS-Simulink Converter 1/1 -> Bus Creator/3  "I_[A]"
  Gain/1 -> Energy_[Wh]/1
  connections:
  PS Gain/RConn1 -- Controlled Current Source/RConn1
  Electrical Reference/LConn1 -- neg_in/RConn1 -- Controlled Current Source/RConn2 -- Voltage Sensor1/RConn2
  power_[W]/RConn1 -- PS Add/LConn2
  PS Constant1/RConn1 -- PS Add/LConn1
  PS Divide/RConn1 -- PS Gain/LConn1
  Voltage Sensor1/RConn1 -- PS Product2/LConn1 -- PS-Simulink Converter 3/LConn1 -- PS Divide/LConn2
  PS Product2/LConn2 -- PS-Simulink Converter 1/LConn1 -- Current Sensor/RConn1
  PS Product2/RConn1 -- PS-Simulink Converter 2/LConn1
  Current Sensor/RConn2 -- Controlled Current Source/LConn1 -- Voltage Sensor1/LConn1
  Current Sensor/LConn1 -- pos_in/RConn1
  PS Add/RConn1 -- PS Divide/LConn1

== system Modell_PADDELEC_RB_V4/MotorController/Speed Controller ==
  V_wref : Inport
  V_w : Inport  Port=2
  200Hz Lowpass Filter : TransferFcn  Denominator=[1/(2*pi*200) 1]
  Messwandler [rpm2volts] : Gain  Gain=5/MotorECU.max_speed
  PID_Speed_Boat : simulink/Continuous/PID Controller  Controller=PI  Form=Parallel  TimeDomain=Continuous-time  UseExternalTs=off  SampleTime=-1  IntegratorMethod=Forward Euler  FilterMethod=Forward Euler  ControllerParametersSource=internal  P=MotorECU.Speed_Prop  I=MotorECU.Speed_Int  D=0  UseFilter=on  N=100  TunerSelectOption=Transfer Function Based (PID Tuner App)  InitialConditionSource=internal  InitialConditionForIntegrator=0  InitialConditionForFilter=0  DifferentiatorICPrevScaledInput=0  ExternalReset=none  TrackingMode=off  Kt=1  LimitOutput=off  UpperSaturationLimit=10  LowerSaturationLimit=-10  LinearizeAsGain=on  AntiWindupMode=none  Kb=1  POutMin=[]  POutMax=[]  IOutMin=[]  IOutMax=[]  DOutMin=[]  DOutMax=[]  NOutMin=[]  NOutMax=[]  SumOutMin=[]  SumOutMax=[]  SaturationOutMin=[]  SaturationOutMax=[]  PParamMin=[]  PParamMax=[]  IParamMin=[]  IParamMax=[]  DParamMin=[]  DParamMax=[]  NParamMin=[]  NParamMax=[]  KbParamMin=[]  KbParamMax=[]  KtParamMin=[]  KtParamMax=[]  KbOutMin=[]  KbOutMax=[]  KtOutMin=[]  KtOutMax=[]  IntegratorOutMin=[]  IntegratorOutMax=[]  FilterOutMin=[]  FilterOutMax=[]  SumI1OutMin=[]  SumI1OutMax=[]  SumI2OutMin=[]  SumI2OutMax=[]  SumI3OutMin=[]  SumI3OutMax=[]  SumI4OutMin=[]  SumI4OutMax=[]  SumDOutMin=[]  SumDOutMax=[]  DifferentiatorOutMin=[]  DifferentiatorOutMax=[]  FilterDiffOutCoefMin=[]  FilterDiffOutCoefMax=[]  ReciprocalOutMin=[]  ReciprocalOutMax=[]  SumDenOutMin=[]  SumDenOutMax=[]  SumNumOutMin=[]  SumNumOutMax=[]  DivideOutMin=[]  DivideOutMax=[]  UdiffTsProdOutMin=[]  UdiffTsProdOutMax=[]  NTsProdOutMin=[]  NTsProdOutMax=[]  UintegralTsProdOutMin=[]  UintegralTsProdOutMax=[]  UngainTsProdOutMin=[]  UngainTsProdOutMax=[]  IntegratorContinuousStateAttributes=''  IntegratorStateMustResolveToSignalObject=off  IntegratorRTWStateStorageClass=Auto  FilterContinuousStateAttributes=''  FilterStateMustResolveToSignalObject=off  FilterRTWStateStorageClass=Auto  ParallelPVariant=InternalParameters  IdealPVariant=Disabled  IVariant=InternalParameters  DVariant=Disabled  IntegratorVariant=Continuous  SatVariant=Disabled  AWVariant=Passthrough  PCopyVariant=Disabled  TRVariant=Disabled  FdbkBlocksVariant=Forward  IdealPFdbkVariant=Disabled  SatFdbkVariant=Disabled  DerivativeFilterVariant=Disabled  NVariant=Disabled  NCopyVariant=Disabled_SignalSpec  FilterICVariant=Disabled  IntegratorICVariant=InternalICs  ExternalResetVariant=Disabled  TRSumVariant=Passthrough  SumFdbkVariant=Disabled  SumVariant=Sum_PI  TsampFilterVariant=InternalTs  TsampNgainVariant=Passthrough  TsampIntegralVariant=Passthrough
  Rate Limiter : RateLimiter  RisingSlewLimit=MotorECU.max_speed/MotorECU.slew_rate_up  FallingSlewLimit=-MotorECU.max_speed/MotorECU.slew_rate_down  SampleTimeMode=inherited
  Sum : Sum  Inputs=+-|
  V_iref : Outport
  wires:
  PID_Speed_Boat/1 -> V_iref/1
  Sum/1 -> PID_Speed_Boat/1
  V_w/1 -> 200Hz Lowpass Filter/1
  V_wref/1 -> Rate Limiter/1
  Rate Limiter/1 -> Messwandler [rpm2volts]/1
  Messwandler [rpm2volts]/1 -> Sum/1
  200Hz Lowpass Filter/1 -> Sum/2

== system Modell_PADDELEC_RB_V4/iPADDLE/MEMS_Data ==
  Beta_Pad : Constant  Value=0
  Bus Creator : BusCreator  Inputs=1
  MEMS : Outport
  wires:
  Beta_Pad/1 -> Bus Creator/1
  Bus Creator/1 -> MEMS/1

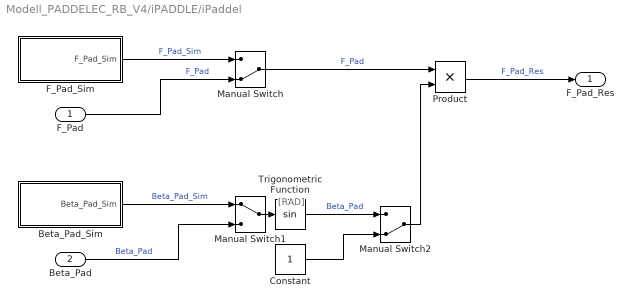
== system Modell_PADDELEC_RB_V4/iPADDLE/iPaddel ==
  note: [RAD]
  F_Pad : Inport
  Beta_Pad : Inport  Port=2
  Beta_Pad_Sim : Subsystem
  Constant : Constant
  F_Pad_Sim : Subsystem
  Manual Switch : ManualSwitch  CurrentSetting=0
  Manual Switch1 : ManualSwitch
  Manual Switch2 : ManualSwitch  CurrentSetting=0
  Product : Product
  Trigonometric Function : Trigonometry
  F_Pad_Res : Outport  VectorParamsAs1DForOutWhenUnconnected=off
  wires:
  F_Pad/1 -> Manual Switch/2  "F_Pad"
  Beta_Pad/1 -> Manual Switch1/2  "Beta_Pad"
  Product/1 -> F_Pad_Res/1  "F_Pad_Res"
  Trigonometric Function/1 -> Manual Switch2/1  "Beta_Pad"
  F_Pad_Sim/1(F_Pad_Sim) -> Manual Switch/1  "F_Pad_Sim"
  Manual Switch/1 -> Product/1  "F_Pad"
  Beta_Pad_Sim/1(Beta_Pad_Sim) -> Manual Switch1/1  "Beta_Pad_Sim"
  Manual Switch1/1 -> Trigonometric Function/1
  Manual Switch2/1 -> Product/2
  Constant/1 -> Manual Switch2/2

== system Modell_PADDELEC_RB_V4/BOAT/Referenzmodell/resistances ==
  v_Boat_In : Inport
  Add : Sum
  Add1 : Sum
  Constant : Constant  Value=0
  Manual Switch : ManualSwitch  CurrentSetting=0
  Manual Switch1 : ManualSwitch
  friction_resistance : Subsystem
  total_resistance : Subsystem
  wave_resistance : Subsystem
  wind_compensation : Subsystem
  F_Resis_Out : Outport  VectorParamsAs1DForOutWhenUnconnected=off
  wires:
  v_Boat_In/1 -> wind_compensation/1(In1), friction_resistance/1(v_Boot), total_resistance/1(In1), wave_resistance/1(v_Boot)
  friction_resistance/1(Fr) -> Add/2
  wave_resistance/1(Fw) -> Add/1
  Add/1 -> Manual Switch/2
  total_resistance/1(Rt) -> Manual Switch/1
  Manual Switch/1 -> Add1/1
  wind_compensation/1(Fr) -> Manual Switch1/1
  Manual Switch1/1 -> Add1/2  "air_resistance"
  Constant/1 -> Manual Switch1/2
  Add1/1 -> F_Resis_Out/1

== system Modell_PADDELEC_RB_V4/MotorController/Current Controller/SL2V_1 ==
  SL : Inport
  Controlled Voltage Source : fl_lib/Electrical/Electrical Sources/Controlled Voltage Source
  Electrical Reference : fl_lib/Electrical/Electrical Elements/Electrical Reference
  Simulink-PS Converter : nesl_utility/Simulink-PS Converter  PhysicalDomain=network_engine_domain  SubClassName=ps_input  LeftPortType=input  RightPortType=output  PseudoPeriodic=off  Frequencies=[]  NoiseDistribution=none  NoiseParameters=[]  Unit=V  AffineConversion=off  FilteringAndDerivatives=zero  SimscapeFilterOrder=1  InputFilterTimeConstant=.001  UdotUserProvided=0
  V : PMIOPort  Side=Right
  wires:
  SL/1 -> Simulink-PS Converter/1
  connections:
  Simulink-PS Converter/RConn1 -- Controlled Voltage Source/RConn1
  V/RConn1 -- Controlled Voltage Source/LConn1
  Electrical Reference/LConn1 -- Controlled Voltage Source/RConn2

== system Modell_PADDELEC_RB_V4/MotorController/Current Controller/SL2V_2 ==
  SL : Inport
  Controlled Voltage Source : fl_lib/Electrical/Electrical Sources/Controlled Voltage Source
  Electrical Reference : fl_lib/Electrical/Electrical Elements/Electrical Reference
  Simulink-PS Converter : nesl_utility/Simulink-PS Converter  PhysicalDomain=network_engine_domain  SubClassName=ps_input  LeftPortType=input  RightPortType=output  PseudoPeriodic=off  Frequencies=[]  NoiseDistribution=none  NoiseParameters=[]  Unit=V  AffineConversion=off  FilteringAndDerivatives=zero  SimscapeFilterOrder=1  InputFilterTimeConstant=.001  UdotUserProvided=0
  V : PMIOPort  Side=Right
  wires:
  SL/1 -> Simulink-PS Converter/1
  connections:
  Electrical Reference/LConn1 -- Controlled Voltage Source/RConn2
  V/RConn1 -- Controlled Voltage Source/LConn1
  Simulink-PS Converter/RConn1 -- Controlled Voltage Source/RConn1

== system Modell_PADDELEC_RB_V4/MotorController/PWM & H-Bridge/PWM Scope ==
  Electrical Reference1 : fl_lib/Electrical/Electrical Elements/Electrical Reference
  PS-Simulink Converter 2 : nesl_utility/PS-Simulink Converter  PhysicalDomain=network_engine_domain  SubClassName=ps_output  LeftPortType=input  RightPortType=output  PseudoPeriodic=off  Frequencies=[]  Unit=V  AffineConversion=off
  REV : Scope
  Voltage Sensor : fl_lib/Electrical/Electrical Sensors/Voltage Sensor
  u : PMIOPort  Side=Left
  wires:
  PS-Simulink Converter 2/1 -> REV/1
  connections:
  Voltage Sensor/RConn2 -- Electrical Reference1/LConn1
  Voltage Sensor/RConn1 -- PS-Simulink Converter 2/LConn1
  u/RConn1 -- Voltage Sensor/LConn1

== system Modell_PADDELEC_RB_V4/MotorController/PWM & H-Bridge/REV Scope ==
  Electrical Reference1 : fl_lib/Electrical/Electrical Elements/Electrical Reference
  PS-Simulink Converter 2 : nesl_utility/PS-Simulink Converter  PhysicalDomain=network_engine_domain  SubClassName=ps_output  LeftPortType=input  RightPortType=output  PseudoPeriodic=off  Frequencies=[]  Unit=V  AffineConversion=off
  REV : Scope
  Voltage Sensor : fl_lib/Electrical/Electrical Sensors/Voltage Sensor
  u : PMIOPort  Side=Left
  wires:
  PS-Simulink Converter 2/1 -> REV/1
  connections:
  u/RConn1 -- Voltage Sensor/LConn1
  Voltage Sensor/RConn1 -- PS-Simulink Converter 2/LConn1
  Voltage Sensor/RConn2 -- Electrical Reference1/LConn1

== system Modell_PADDELEC_RB_V4/iPADDLE/iPaddel/Beta_Pad_Sim ==
  Add : Sum
  "Beta_Pad_Sim " : Sin  Amplitude=45  Frequency=3  SampleTime=0
  Constant : Constant  Value=0
  Constant1 : Constant  Value=45
  Gain : Gain  Gain=pi/180
  Switch : Switch
  Beta_Pad_Sim : Outport
  wires:
  Constant/1 -> Switch/3
  Gain/1 -> Beta_Pad_Sim/1
  "Beta_Pad_Sim "/1 -> Switch/2, Switch/1
  Switch/1 -> Add/1
  Add/1 -> Gain/1
  Constant1/1 -> Add/2

== system Modell_PADDELEC_RB_V4/iPADDLE/iPaddel/F_Pad_Sim ==
  Constant : Constant  Value=0
  "F_Pad_Sim " : Sin  Amplitude=80  Frequency=3  SampleTime=0
  Switch : Switch
  F_Pad_Sim : Outport
  wires:
  "F_Pad_Sim "/1 -> Switch/2, Switch/1
  Switch/1 -> F_Pad_Sim/1
  Constant/1 -> Switch/3

== system Modell_PADDELEC_RB_V4/BOAT/Referenzmodell/resistances/friction_resistance ==
  v_Boot : Inport
  A_s : Constant  Value=A_s
  Math Function : Math  Operator=square  SignedPower=on  SaturateOnIntegerOverflow=on
  Product : Product  Inputs=4
  Roh/2 : Constant  Value=997/2
  c_r : Constant  Value=c_r
  Fr : Outport  VectorParamsAs1DForOutWhenUnconnected=off
  wires:
  v_Boot/1 -> Math Function/1
  Product/1 -> Fr/1
  c_r/1 -> Product/3
  A_s/1 -> Product/2
  Roh/2/1 -> Product/1
  Math Function/1 -> Product/4

== system Modell_PADDELEC_RB_V4/BOAT/Referenzmodell/resistances/total_resistance ==
  In1 : Inport
  Fcn : Fcn  Expr=-2.9119*u^5+28.358*u^4-99.765*u^3+165.24*u^2-119.06*u+33.315
  Rt : Outport
  wires:
  In1/1 -> Fcn/1
  Fcn/1 -> Rt/1

== system Modell_PADDELEC_RB_V4/BOAT/Referenzmodell/resistances/wave_resistance ==
  v_Boot : Inport
  Fcn : Fcn  Expr=5*u*exp(u/(1.25*(4^0.5)))
  Fw : Outport
  wires:
  v_Boot/1 -> Fcn/1
  Fcn/1 -> Fw/1

== system Modell_PADDELEC_RB_V4/BOAT/Referenzmodell/resistances/wind_compensation ==
  In1 : Inport
  A_s : Constant  Value=0.54
  Add : Sum
  Math Function : Math  Operator=square  SignedPower=on  SaturateOnIntegerOverflow=on
  Product : Product  Inputs=4
  Roh/2 : Constant  Value=1.269/2
  c_r : Constant  Value=0.8
  wind_speed : Constant  Value=4.5
  Fr : Outport  VectorParamsAs1DForOutWhenUnconnected=off
  wires:
  Math Function/1 -> Product/4
  Roh/2/1 -> Product/1
  A_s/1 -> Product/2
  c_r/1 -> Product/3
  Product/1 -> Fr/1
  wind_speed/1 -> Add/2
  In1/1 -> Add/1
  Add/1 -> Math Function/1
